simulink model "matlabfun_cancella"  (R2020b)
settings: Solver=VariableStepAuto  StartTime=0.0  StopTime=10.0  RelTol=1e-3
settings Model: Creator=Matteo  LastModifiedBy=Matteo

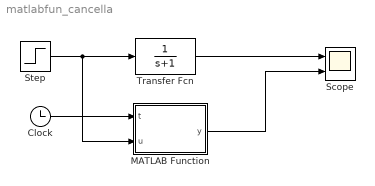
== system matlabfun_cancella ==
  Clock : Clock
  MATLAB Function : MATLAB Function  TreatAsAtomicUnit=on
  Scope : Scope  NumInputPorts=2
  Step : Step  Time=0  SampleTime=0
  Transfer Fcn : TransferFcn  Denominator=[1 1]
  wires:
  Step/1 -> MATLAB Function/2(u), Transfer Fcn/1
  MATLAB Function/1(y) -> Scope/2
  Transfer Fcn/1 -> Scope/1
  Clock/1 -> MATLAB Function/1(t)

== matlab function matlabfun_cancella/MATLAB Function ==
  data: t input; u input; y output
function y = fcn(t,u)



y = (1-exp(-t))*u;
